simulink model "Model3"  (R2020a)
settings: Solver=FixedStepAuto  StartTime=0.0  StopTime=10.0  FixedStep=0.001  MaxStep=0.2  RelTol=1e-3
model workspace (MAT data in the model file):
  C = 18
  R = 16
libraries: simulink x2
settings Model: Creator=HP  LastModifiedBy=HP

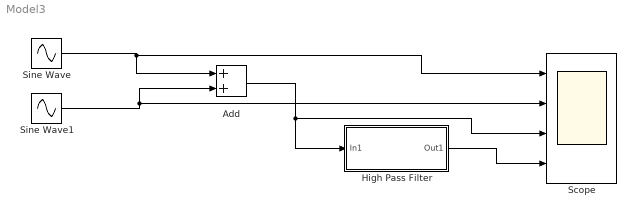
== system Model3 ==
  Add : Sum
  High Pass Filter : Subsystem
  Scope : Scope  NumInputPorts=4
  Sine Wave : Sin  Amplitude=50  SampleTime=0
  Sine Wave1 : Sin  Amplitude=5  Frequency=10  SampleTime=0
  wires:
  Sine Wave/1 -> Scope/1, Add/1
  Sine Wave1/1 -> Scope/2, Add/2
  Add/1 -> High Pass Filter/1(In1), Scope/3
  High Pass Filter/1(Out1) -> Scope/4

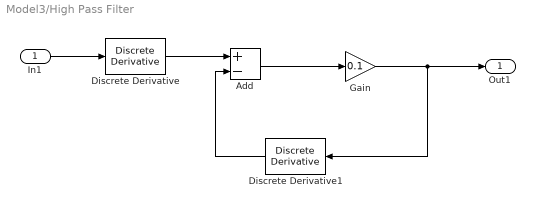
== system Model3/High Pass Filter ==
  In1 : Inport
  Add : Sum  Inputs=+-
  Discrete Derivative : simulink/Discrete/Discrete Derivative  gainval=1.0  ICPrevScaledInput=0.0  OutMin=[]  OutMax=[]  OutDataType=fixdt(1, 16)  OutScaling=2^-10  DoSatur=off
  Discrete Derivative1 : simulink/Discrete/Discrete Derivative  gainval=1.0  ICPrevScaledInput=0.0  OutMin=[]  OutMax=[]  OutDataType=fixdt(1, 16)  OutScaling=2^-10  DoSatur=off
  Gain : Gain  Gain=0.1
  Out1 : Outport
  wires:
  Discrete Derivative/1 -> Add/1
  In1/1 -> Discrete Derivative/1
  Add/1 -> Gain/1
  Gain/1 -> Discrete Derivative1/1, Out1/1
  Discrete Derivative1/1 -> Add/2
